simulink model "Solar_Seguidor_V2"  (R2021b)
settings: Solver=ode1  StartTime=0.0  StopTime=10  FixedStep=25e-6  RelTol=1e-3
PostLoadFcn:
  | %clc; clear all; close all;
  | %%%%%%%%%%%%%%%%%%%%%%%%%%%%%%%%%%%%%%%%%%%%%%%%
  | %%%%%%%%% Solar seguidor de rede %%%%%%%%%%
  | %%%%%%%%%%%%%%%%%%%%%%%%%%%%%%%%%%%%%%%%%%%%%%%%
  | %%%% Nominal Parameters %%%%
  | Pnom = 16e3;                                         % Potencia Nominal
  | Vnom_rms = 210;                                    % V linha rms
  | Vnom_peak = sqrt(2/3)*Vnom_rms;                     % V fase pico
  | FP_min = 1;                                       % Para suporte de reativo
  | Snom = Pnom/FP_min;                                 % Potencia aparente
  | Irms = Pnom/(sqrt(3)*Vnom_rms);                     % Ig rms
  | Inom_peak = Irms*sqrt(2);                           % Ig pico
  | Zbase = Vnom_peak/Inom_peak;                        % Impedancia Base
  | f = 60;                                             % Freq nominal
  | wnom = 2*pi*60;                                     % Freq Ang. nominal
  | m = 0.805;                                            % Indice mod nominal
  | Vdc = 2*(Vnom_peak/m);                              % Vcc
  | Vdc_2 = Vdc/2;                                      % Metade Vcc
  | Kconv = Zbase;                                      % Ganho conversor
  | %%%% Transformer %%%%
  | S_trafo = 250e3;                                      % transformer apparent power
  | Vrms_high = 400;                                   % transformer secondary voltage - Wye connection
  | Vrms_low = 210;                                   % transformer primary voltage - Delta connection
  | N = Vrms_high/Vrms_low;                             % transformation relationship
  | X_pu_trafo = 0.03;                                 % transformer p.u. reactance
  | Zb_trafo_high = ((Vrms_high)^2)/S_trafo;            % secondary base impedance
  | Zb_trafo = ((Vnom_rms)^2)/S_trafo;                  % primary base impedance
  | L_trafo = (X_pu_trafo*Zb_trafo)/wnom;               % primary inductance
  | %%%% LCL Filter Project %%%%
  | fsw = 105*60;%105*60;                                         % switching frequency
  | ripple = 0.05;                                       % current ripple
  | L1 = Vdc/(6*ripple*Inom_peak*fsw);                  % inductor L1
  |  RL1 = 0.005;                                        % L1 resistance
  |  Cbase = 1/(wnom*Kconv);                             % base capacitance
  |  Cf = 0.05*Cbase;                                    % filter capacitor
  | % Calculo do filtro
  | Sbase = 16e3;
  | %Sbase = 200e3*1.12;
  | V_LL = 210;
  | V_LG = 210/sqrt(3);
  | Vbase = V_LG*sqrt(2);
  | Ibase = (Sbase*sqrt(2))/(V_LG*3)*sqrt(3/2);
  | Zbase = (V_LL^2)/Sbase;
  | Rbase = Zbase;
  | Xbase = Zbase;
  | Lbase = Xbase/(2*pi*60);
  | Cbase = 1/(Xbase*2*pi*60);
  | w = 2*pi*60;
  | Q = 70;
  | Lf = 0.15*Lbase;
  | Cf = 0.05*Cbase;
  | fc = 1/(2*pi*sqrt(Lf*Cf));
  | R = (w*Lf)/Q;
  | Lf = L1;
  | R = RL1;
  | ka=0.2;                                             % attenuation factor
  | L2 = (sqrt(1/(ka^2))+1)/(Cf*((2*pi*fsw)^2));        % inductor L2
  | RL2 = 0.005;                                        % L2 resistance
  | w_res = sqrt((L1+L2+L_trafo)/(L1*L2*Cf));           % resonant angular frequency
  | f_res = w_res/(2*pi);                               % resonant frequency
  | ... (+31 lines)
InitFcn:
  | %clc; clear all; close all;
  | %%%%%%%%%%%%%%%%%%%%%%%%%%%%%%%%%%%%%%%%%%%%%%%%
  | %%%%%%%%% Solar seguidor de rede %%%%%%%%%%
  | %%%%%%%%%%%%%%%%%%%%%%%%%%%%%%%%%%%%%%%%%%%%%%%%
  | %%%% Nominal Parameters %%%%
  | Pnom = 16e3;                                         % Potencia Nominal
  | Vnom_rms = 210;                                    % V linha rms
  | Vnom_peak = sqrt(2/3)*Vnom_rms;                     % V fase pico
  | FP_min = 1;                                       % Para suporte de reativo
  | Snom = Pnom/FP_min;                                 % Potencia aparente
  | Irms = Pnom/(sqrt(3)*Vnom_rms);                     % Ig rms
  | Inom_peak = Irms*sqrt(2);                           % Ig pico
  | Zbase = Vnom_peak/Inom_peak;                        % Impedancia Base
  | f = 60;                                             % Freq nominal
  | wnom = 2*pi*60;                                     % Freq Ang. nominal
  | m = 0.805;                                            % Indice mod nominal
  | Vdc = 2*(Vnom_peak/m);                              % Vcc
  | Vdc_2 = Vdc/2;                                      % Metade Vcc
  | Kconv = Zbase;                                      % Ganho conversor
  | %%%% Transformer %%%%
  | S_trafo = 250e3;                                      % transformer apparent power
  | Vrms_high = 400;                                   % transformer secondary voltage - Wye connection
  | Vrms_low = 210;                                   % transformer primary voltage - Delta connection
  | N = Vrms_high/Vrms_low;                             % transformation relationship
  | X_pu_trafo = 0.03;                                 % transformer p.u. reactance
  | Zb_trafo_high = ((Vrms_high)^2)/S_trafo;            % secondary base impedance
  | Zb_trafo = ((Vnom_rms)^2)/S_trafo;                  % primary base impedance
  | L_trafo = (X_pu_trafo*Zb_trafo)/wnom;               % primary inductance
  | %%%% LCL Filter Project %%%%
  | fsw = 105*60;%105*60;                                         % switching frequency
  | ripple = 0.05;                                       % current ripple
  | L1 = Vdc/(6*ripple*Inom_peak*fsw);                  % inductor L1
  |  RL1 = 0.005;                                        % L1 resistance
  |  Cbase = 1/(wnom*Kconv);                             % base capacitance
  |  Cf = 0.05*Cbase;                                    % filter capacitor
  | % Calculo do filtro
  | Sbase = 16e3;
  | %Sbase = 200e3*1.12;
  | V_LL = 210;
  | V_LG = 210/sqrt(3);
  | Vbase = V_LG*sqrt(2);
  | Ibase = (Sbase*sqrt(2))/(V_LG*3)*sqrt(3/2);
  | Zbase = (V_LL^2)/Sbase;
  | Rbase = Zbase;
  | Xbase = Zbase;
  | Lbase = Xbase/(2*pi*60);
  | Cbase = 1/(Xbase*2*pi*60);
  | w = 2*pi*60;
  | Q = 70;
  | Lf = 0.15*Lbase;
  | Cf = 0.05*Cbase;
  | fc = 1/(2*pi*sqrt(Lf*Cf));
  | R = (w*Lf)/Q;
  | Lf = L1;
  | R = RL1;
  | ka=0.2;                                             % attenuation factor
  | L2 = (sqrt(1/(ka^2))+1)/(Cf*((2*pi*fsw)^2));        % inductor L2
  | RL2 = 0.005;                                        % L2 resistance
  | w_res = sqrt((L1+L2+L_trafo)/(L1*L2*Cf));           % resonant angular frequency
  | f_res = w_res/(2*pi);                               % resonant frequency
  | ... (+31 lines)
undefined symbols (not defined in the file): D1, Delta, DERS_models, DiscIntNeverNeededParam, eHS, I, Ia_PV, Ib_PV, Ic_PV, Left, parameter_set_id, ph, PV_system, type, V, Va_grid, Vb_grid, Vc_grid
libraries: powerlib_meascontrol x17, rtlab x14, spsThreePhaseSeriesRLCBranchLib x9, spsCurrentMeasurementLib x9, artemis x7, spsThreePhaseVIMeasurementLib x6, slpidlib x6, rteventslib x6, spsabctodq0Lib x4, spsThreePhaseTransformerTwoWindingsLib x3, simulink x3, spsPVArrayLib x3
(part 3 of 4)

== system Solar_Seguidor_V2/SM_mestre1/PV_system/Subsystem1/THD ==
  Iabc : Inport
  Demux : Demux  Outputs=3
  Gain1 : Gain  Gain=100
  Gain2 : Gain  Gain=100
  Gain3 : Gain  Gain=100
  Mux : Mux  Inputs=3
  Saturation : Saturate  UpperLimit=7
  Saturation1 : Saturate  UpperLimit=7
  Saturation2 : Saturate  UpperLimit=7
  THD : powerlib_meascontrol/Measurements/THD  Freq=60  Ts=Ts
  THD1 : powerlib_meascontrol/Measurements/THD  Freq=60  Ts=Ts
  THD2 : powerlib_meascontrol/Measurements/THD  Freq=60  Ts=Ts
  THD_I : Outport
  wires:
  Demux/1 -> THD/1
  Saturation2/1 -> Mux/3
  Saturation/1 -> Mux/1
  THD/1 -> Gain1/1
  Saturation1/1 -> Mux/2
  Demux/3 -> THD2/1
  THD1/1 -> Gain2/1
  Gain2/1 -> Saturation1/1
  Gain3/1 -> Saturation2/1
  THD2/1 -> Gain3/1
  Demux/2 -> THD1/1
  Gain1/1 -> Saturation/1
  Iabc/1 -> Demux/1
  Mux/1 -> THD_I/1

== system Solar_Seguidor_V2/SM_mestre1/PV_system/VSC_Control/Current Controller ==
  note: Current Controller (with feedforward)
  VdVq_mes : Inport  PortDimensions=2
  IdIq_mes : Inport  Port=2  PortDimensions=2
  IdIq_ref : Inport  Port=3  PortDimensions=2
  hab : Inport  Port=4
  Add1 : Sum  Inputs=+-
  Add2 : Sum
  Add3 : Sum
  Demux : Demux  Outputs=2
  Demux1 : Demux  Outputs=2
  Mux : Mux  Inputs=2
  Mux1 : Mux  Inputs=2
  PI : slpidlib/PID Controller  Controller=PI  Form=Parallel  TimeDomain=Continuous-time  UseExternalTs=off  SampleTime=Ts  IntegratorMethod=Forward Euler  FilterMethod=Forward Euler  ControllerParametersSource=internal  P=kp_current_pu  I=ki_current_pu  D=0  UseFilter=on  N=100  TunerSelectOption=Transfer Function Based (PID Tuner App)  InitialConditionSource=internal  InitialConditionForIntegrator=0  InitialConditionForFilter=0  DifferentiatorICPrevScaledInput=0  ExternalReset=rising  TrackingMode=off  Kt=1  LimitOutput=off  SatLimitsSource=internal  UpperSaturationLimit=2  LowerSaturationLimit=-2  LinearizeAsGain=off  AntiWindupMode=none  Kb=1  POutMin=[]  POutMax=[]  IOutMin=[]  IOutMax=[]  DOutMin=[]  DOutMax=[]  NOutMin=[]  NOutMax=[]  SumOutMin=[]  SumOutMax=[]  SaturationOutMin=[]  SaturationOutMax=[]  PParamMin=[]  PParamMax=[]  IParamMin=[]  IParamMax=[]  DParamMin=[]  DParamMax=[]  NParamMin=[]  NParamMax=[]  KbParamMin=[]  KbParamMax=[]  KtParamMin=[]  KtParamMax=[]  KbOutMin=[]  KbOutMax=[]  KtOutMin=[]  KtOutMax=[]  IntegratorOutMin=[]  IntegratorOutMax=[]  FilterOutMin=[]  FilterOutMax=[]  SumI1OutMin=[]  SumI1OutMax=[]  SumI2OutMin=[]  SumI2OutMax=[]  SumI3OutMin=[]  SumI3OutMax=[]  SumI4OutMin=[]  SumI4OutMax=[]  SumDOutMin=[]  SumDOutMax=[]  DifferentiatorOutMin=[]  DifferentiatorOutMax=[]  FilterDiffOutCoefMin=[]  FilterDiffOutCoefMax=[]  ReciprocalOutMin=[]  ReciprocalOutMax=[]  SumDenOutMin=[]  SumDenOutMax=[]  SumNumOutMin=[]  SumNumOutMax=[]  DivideOutMin=[]  DivideOutMax=[]  UdiffTsProdOutMin=[]  UdiffTsProdOutMax=[]  NTsProdOutMin=[]  NTsProdOutMax=[]  UintegralTsProdOutMin=[]  UintegralTsProdOutMax=[]  UngainTsProdOutMin=[]  UngainTsProdOutMax=[]  IntegratorContinuousStateAttributes=''  IntegratorStateMustResolveToSignalObject=off  IntegratorRTWStateStorageClass=Auto  FilterContinuousStateAttributes=''  FilterStateMustResolveToSignalObject=off  FilterRTWStateStorageClass=Auto  ParallelPVariant=InternalParameters  IdealPVariant=Disabled  IVariant=InternalParameters  DVariant=Disabled  IntegratorVariant=Continuous  SatVariant=Disabled  AWVariant=Passthrough  PCopyVariant=Disabled  TRVariant=Disabled  FdbkBlocksVariant=Forward  IdealPFdbkVariant=Disabled  SatFdbkVariant=Disabled  DerivativeFilterVariant=Disabled  NVariant=Disabled  NCopyVariant=Disabled_SignalSpec  FilterICVariant=Disabled  IntegratorICVariant=InternalICs  ExternalResetVariant=ExternalReset  TRSumVariant=Passthrough  SumFdbkVariant=Disabled  SumVariant=Sum_PI  TsampFilterVariant=InternalTs  TsampNgainVariant=Passthrough  TsampIntegralVariant=Passthrough  ExternalSaturationOutDataTypeStr=Inherit: Same as second input
  Product : Product
  Saturation : Saturate  UpperLimit=10  LowerLimit=-10
  Sum : Sum  Inputs=|+-
  wL : Gain  Gain=decouple_pu  SaturateOnIntegerOverflow=on  OutDataTypeStr=Inherit: Same as input  ParamDataTypeStr=Inherit: Same as input
  wL2 : Gain  Gain=decouple_pu  SaturateOnIntegerOverflow=on  OutDataTypeStr=Inherit: Same as input  ParamDataTypeStr=Inherit: Same as input
  m_dq : Outport  VectorParamsAs1DForOutWhenUnconnected=off
  wires:
  wL/1 -> Add1/2
  Mux/1 -> Add2/2
  PI/1 -> Add2/1  "PI"
  Sum/1 -> PI/1
  Saturation/1 -> m_dq/1
  VdVq_mes/1 -> Demux/1
  Demux/1 -> Add1/1
  Demux1/1 -> wL2/1
  Demux1/2 -> wL/1
  wL2/1 -> Add3/2
  Add1/1 -> Mux/1
  Demux/2 -> Add3/1
  Add3/1 -> Mux/2
  Add2/1 -> Product/1
  Product/1 -> Saturation/1
  hab/1 -> [hab]
  [hab] -> PI/2
  [hab] -> Product/2
  Mux1/1 -> [Idq_scope]
  IdIq_ref/1 -> Mux1/1, Sum/1
  IdIq_mes/1 -> Mux1/2, Sum/2, Demux1/1

== system Solar_Seguidor_V2/SM_mestre1/PV_system/VSC_Control/Maximum Power Point ==
  Vpv : Inport
  Ipv : Inport  Port=2
  Enable_MPPT : Inport  Port=3
  Constant : Constant  Value=Vdc
  MPPT Parameters : Subsystem
  MPPT Controller using Perturbe & Observe technique 2 : MATLAB Function  TreatAsAtomicUnit=on
  Switch1 : Switch
  ZOH/4 : ZeroOrderHold  SampleTime=Ts_Control
  ZOH/6 : ZeroOrderHold  SampleTime=Ts_Control
  Gmpp : Outport
  wires:
  Ipv/1 -> ZOH/6/1
  Vpv/1 -> ZOH/4/1
  ZOH/4/1 -> MPPT Controller using Perturbe & Observe technique 2/3(V)
  ZOH/6/1 -> MPPT Controller using Perturbe & Observe technique 2/4(I)
  MPPT Parameters/1(Param) -> MPPT Controller using Perturbe & Observe technique 2/1(Param)
  Enable_MPPT/1 -> MPPT Controller using Perturbe & Observe technique 2/2(Enabled), Switch1/2
  Constant/1 -> Switch1/3
  Switch1/1 -> Gmpp/1
  MPPT Controller using Perturbe & Observe technique 2/1(D) -> Switch1/1

== system Solar_Seguidor_V2/SM_mestre1/PV_system/VSC_Control/PLL & dq ==
  Vabc : Inport
  Iabc : Inport  Port=2
  Demux : Demux  Outputs=2
  I_to_pu : Gain  Gain=1/(Ibase*1.15)  SaturateOnIntegerOverflow=on  OutDataTypeStr=Inherit: Same as input  ParamDataTypeStr=Inherit: Same as input
  Iabc_PV : Scope
  Iabc_PV_pu : Scope
  Idq : Scope
  Mux1 : Mux  Inputs=2
  PLL (3ph) : powerlib_meascontrol/PLL/PLL (3ph)  Fmin=45  Par_Init="[-0.57  60]"  ParK=[180, 3200, 1]  TcD=Ts_Control  MaxRateChangeFreq=12  FilterCutOffFreq=25  Ts=Ts_Control  AGC=on
  Scope : Scope
  Scope1 : Scope
  Selector1 : Selector  InputPortWidth=3  IndexOptions=Index vector (dialog)  Indices=[1 2]  OutputSizes=1
  Selector2 : Selector  InputPortWidth=3  IndexOptions=Index vector (dialog)  Indices=[1 2]  OutputSizes=1
  Subsystem : Subsystem
  Transfer Fcn1 : TransferFcn  Denominator=[2.53e-4 1]
  Transfer Fcn4 : TransferFcn  Denominator=[2.53e-4 1]
  V_to_pu : Gain  Gain=1/(400*sqrt(2)/sqrt(3))  SaturateOnIntegerOverflow=on  OutDataTypeStr=Inherit: Same as input  ParamDataTypeStr=Inherit: Same as input
  abc to dq0 : powerlib_meascontrol/Transformations/abc to dq0  Alignment=90 degrees behind phase A axis
  abc to dq1 : powerlib_meascontrol/Transformations/abc to dq0  Alignment=90 degrees behind phase A axis
  P_PV : Outport
  Freq : Outport  Port=2
  wt : Outport  Port=3  VectorParamsAs1DForOutWhenUnconnected=off
  VdVq : Outport  Port=4  VectorParamsAs1DForOutWhenUnconnected=off
  IdIq : Outport  Port=5  VectorParamsAs1DForOutWhenUnconnected=off
  wires:
  Iabc/1 -> Iabc_PV/1, Subsystem/3(Iabc), I_to_pu/1
  I_to_pu/1 -> Iabc_PV_pu/1, abc to dq1/1
  V_to_pu/1 -> abc to dq0/1, PLL (3ph)/1
  abc to dq1/1 -> Selector1/1
  Vabc/1 -> Subsystem/2(Vabc), V_to_pu/1
  abc to dq0/1 -> Selector2/1
  PLL (3ph)/1 -> Scope1/1, Freq/1
  Selector1/1 -> Demux/1
  Demux/1 -> Transfer Fcn4/1
  Demux/2 -> Transfer Fcn1/1
  Mux1/1 -> Idq/1, IdIq/1
  Selector2/1 -> Scope/1, VdVq/1
  Subsystem/1(P_PV) -> P_PV/1
  PLL (3ph)/2 -> Subsystem/1(wt), abc to dq1/2, abc to dq0/2, wt/1
  Transfer Fcn4/1 -> Mux1/1
  Transfer Fcn1/1 -> Mux1/2

== system Solar_Seguidor_V2/SM_mestre1/PV_system/VSC_Control/PWM ==
  Uabc_ref : Inport
  Constant10 : Constant  Value=2
  Constant11 : Constant  Value=3*35*60
  Constant9 : Constant
  Demux8 : Demux  Outputs=3
  Divide7 : Product  Inputs=*/
  Divide8 : Product  Inputs=*/
  Divide9 : Product  Inputs=*/
  Mux11 : Mux  Inputs=3
  Mux12 : Mux  Inputs=2
  RTE Conversion1 : rteventslib/Signal Attributes/RTE Conversion  inputdatatype=RTE Boolean  outputdatatype=Double  compensation=Enabled  nbMaxEvents=4  sampleTime=Ts
  RTE SPWM1 : rteventslib/Sources/RTE SPWM  NumberPhases=3-ph  CenterAlignmentMode=On  MaxFreq=inf  MinFreq=0  EnablingPort=off  ComplementaryMode=on  SpaceVector=off  RiseTimeDelay=0  MaxEvents=4  SampleTime=Ts
  Saturation : Saturate  UpperLimit=2  LowerLimit=-2
  Scope : Scope
  Scope8 : Scope
  Selector1 : Selector  InputPortWidth=6  IndexOptions=Index vector (dialog)  Indices=[1 4 2 5 3 6]  OutputSizes=1
  Sum16 : Sum  Inputs=|++
  Sum17 : Sum  Inputs=|++
  Sum18 : Sum  Inputs=|++
  Uref : Outport  VectorParamsAs1DForOutWhenUnconnected=off
  wires:
  RTE Conversion1/1 -> Selector1/1
  Mux12/1 -> RTE Conversion1/1
  Demux8/3 -> Sum18/1
  Demux8/1 -> Sum16/1
  Divide7/1 -> Mux11/1
  Mux11/1 -> Scope8/1, RTE SPWM1/2
  Sum18/1 -> Divide9/1
  Divide8/1 -> Mux11/2
  Demux8/2 -> Sum17/1
  Uabc_ref/1 -> Saturation/1
  RTE SPWM1/2 -> Mux12/2
  Divide9/1 -> Mux11/3
  Sum17/1 -> Divide8/1
  Constant10/1 -> Divide7/2, Divide8/2, Divide9/2
  Sum16/1 -> Divide7/1
  Constant11/1 -> RTE SPWM1/1
  Selector1/1 -> Uref/1
  Constant9/1 -> Sum16/2, Sum17/2, Sum18/2
  RTE SPWM1/1 -> Mux12/1
  Saturation/1 -> Scope/1, Demux8/1

== system Solar_Seguidor_V2/SM_mestre1/PV_system/VSC_Control/Uabc_ref Generation  ==
  note: Uabc_ref Generation
  wt : Inport
  m_dq : Inport  Port=2
  Constant5 : Constant  Value=0
  Mux : Mux  Inputs=2
  Scope : Scope
  dq0 to abc : spsdq0toabcLib/dq0 to abc  Alignment=90 degrees behind phase A axis
  Uabc_ref : Outport  VectorParamsAs1DForOutWhenUnconnected=off
  wires:
  Mux/1 -> dq0 to abc/1
  Constant5/1 -> Mux/2
  wt/1 -> dq0 to abc/2
  dq0 to abc/1 -> Uabc_ref/1
  m_dq/1 -> Scope/1, Mux/1

== system Solar_Seguidor_V2/SM_mestre1/PV_system/VSC_Control/Voltage DC Controller ==
  note: Voltage Controller
  Vdc_mes : Inport  PortDimensions=1
  Vdc_ref : Inport  Port=2  PortDimensions=1
  hab : Inport  Port=3
  Id_refm : Scope
  Math Function1 : Math  Operator=square  SaturateOnIntegerOverflow=on
  Math Function2 : Math  Commented=on  Operator=square  SaturateOnIntegerOverflow=on
  Math Function3 : Math  Operator=square  SaturateOnIntegerOverflow=on
  Mux : Mux  Inputs=2
  PI : slpidlib/PID Controller  Controller=PI  Form=Parallel  TimeDomain=Continuous-time  UseExternalTs=off  SampleTime=Ts  IntegratorMethod=Trapezoidal  FilterMethod=Forward Euler  ControllerParametersSource=internal  P=Kp_dc  I=ki_dc_pu  D=0  UseFilter=on  N=100  TunerSelectOption=Transfer Function Based (PID Tuner App)  InitialConditionSource=internal  InitialConditionForIntegrator=0  InitialConditionForFilter=0  DifferentiatorICPrevScaledInput=0  ExternalReset=rising  TrackingMode=off  Kt=1  LimitOutput=on  SatLimitsSource=internal  UpperSaturationLimit=1.4  LowerSaturationLimit=-2  LinearizeAsGain=off  AntiWindupMode=clamping  Kb=1  POutMin=[]  POutMax=[]  IOutMin=[]  IOutMax=[]  DOutMin=[]  DOutMax=[]  NOutMin=[]  NOutMax=[]  SumOutMin=[]  SumOutMax=[]  SaturationOutMin=[]  SaturationOutMax=[]  PParamMin=[]  PParamMax=[]  IParamMin=[]  IParamMax=[]  DParamMin=[]  DParamMax=[]  NParamMin=[]  NParamMax=[]  KbParamMin=[]  KbParamMax=[]  KtParamMin=[]  KtParamMax=[]  KbOutMin=[]  KbOutMax=[]  KtOutMin=[]  KtOutMax=[]  IntegratorOutMin=[]  IntegratorOutMax=[]  FilterOutMin=[]  FilterOutMax=[]  SumI1OutMin=[]  SumI1OutMax=[]  SumI2OutMin=[]  SumI2OutMax=[]  SumI3OutMin=[]  SumI3OutMax=[]  SumI4OutMin=[]  SumI4OutMax=[]  SumDOutMin=[]  SumDOutMax=[]  DifferentiatorOutMin=[]  DifferentiatorOutMax=[]  FilterDiffOutCoefMin=[]  FilterDiffOutCoefMax=[]  ReciprocalOutMin=[]  ReciprocalOutMax=[]  SumDenOutMin=[]  SumDenOutMax=[]  SumNumOutMin=[]  SumNumOutMax=[]  DivideOutMin=[]  DivideOutMax=[]  UdiffTsProdOutMin=[]  UdiffTsProdOutMax=[]  NTsProdOutMin=[]  NTsProdOutMax=[]  UintegralTsProdOutMin=[]  UintegralTsProdOutMax=[]  UngainTsProdOutMin=[]  UngainTsProdOutMax=[]  IntegratorContinuousStateAttributes=''  IntegratorStateMustResolveToSignalObject=off  IntegratorRTWStateStorageClass=Auto  FilterContinuousStateAttributes=''  FilterStateMustResolveToSignalObject=off  FilterRTWStateStorageClass=Auto  ParallelPVariant=InternalParameters  IdealPVariant=Disabled  IVariant=InternalParameters  DVariant=Disabled  IntegratorVariant=Continuous  SatVariant=Enabled  AWVariant=ContClampingParallel  PCopyVariant=Disabled  TRVariant=Disabled  FdbkBlocksVariant=Forward  IdealPFdbkVariant=Disabled  SatFdbkVariant=Disabled  DerivativeFilterVariant=Disabled  NVariant=Disabled  NCopyVariant=Disabled_SignalSpec  FilterICVariant=Disabled  IntegratorICVariant=InternalICs  ExternalResetVariant=ExternalReset  TRSumVariant=Passthrough  SumFdbkVariant=Disabled  SumVariant=Sum_PI  TsampFilterVariant=InternalTs  TsampNgainVariant=Passthrough  TsampIntegralVariant=Passthrough  ExternalSaturationOutDataTypeStr=Inherit: Same as second input
  Rtot_pu1 : Gain  Gain=1/430  SaturateOnIntegerOverflow=on  OutDataTypeStr=Inherit: Same as input  ParamDataTypeStr=Inherit: Same as input
  Rtot_pu2 : Gain  Gain=1/430  SaturateOnIntegerOverflow=on  OutDataTypeStr=Inherit: Same as input  ParamDataTypeStr=Inherit: Same as input
  Rtot_pu3 : Gain  Gain=-1  SaturateOnIntegerOverflow=on  OutDataTypeStr=Inherit: Same as input  ParamDataTypeStr=Inherit: Same as input
  Saturation : Saturate  UpperLimit=1.2  LowerLimit=0
  Sum : Sum  Inputs=|-+
  Transfer Fcn2 : TransferFcn  Commented=on  Denominator=[2.53e-4 1]
  Id_ref : Outport  SampleTime=Ts  InitialOutput=0  VectorParamsAs1DForOutWhenUnconnected=off
  wires:
  Rtot_pu3/1 -> PI/1
  Vdc_ref/1 -> Rtot_pu2/1
  Sum/1 -> Rtot_pu3/1
  hab/1 -> PI/2
  Mux/1 -> [Vdc_scope]
  Rtot_pu1/1 -> Mux/1, Math Function1/1
  Rtot_pu2/1 -> Mux/2, Math Function3/1
  Math Function1/1 -> Sum/1
  Math Function3/1 -> Sum/2
  PI/1 -> Id_refm/1, Saturation/1
  Vdc_mes/1 -> Rtot_pu1/1
  Saturation/1 -> Id_ref/1

== system Solar_Seguidor_V2/SM_mestre1/PV_system1/Subsystem1/THD ==
  Iabc : Inport
  Demux : Demux  Outputs=3
  Gain1 : Gain  Gain=100
  Gain2 : Gain  Gain=100
  Gain3 : Gain  Gain=100
  Mux : Mux  Inputs=3
  Saturation : Saturate  UpperLimit=7
  Saturation1 : Saturate  UpperLimit=7
  Saturation2 : Saturate  UpperLimit=7
  THD : powerlib_meascontrol/Measurements/THD  Freq=60  Ts=Ts
  THD1 : powerlib_meascontrol/Measurements/THD  Freq=60  Ts=Ts
  THD2 : powerlib_meascontrol/Measurements/THD  Freq=60  Ts=Ts
  THD_I : Outport
  wires:
  Mux/1 -> THD_I/1
  Iabc/1 -> Demux/1
  Gain1/1 -> Saturation/1
  Demux/2 -> THD1/1
  THD2/1 -> Gain3/1
  Gain3/1 -> Saturation2/1
  Gain2/1 -> Saturation1/1
  THD1/1 -> Gain2/1
  Demux/3 -> THD2/1
  Saturation1/1 -> Mux/2
  THD/1 -> Gain1/1
  Saturation/1 -> Mux/1
  Saturation2/1 -> Mux/3
  Demux/1 -> THD/1

== system Solar_Seguidor_V2/SM_mestre1/PV_system1/VSC_Control/Current Controller ==
  note: Current Controller (with feedforward)
  VdVq_mes : Inport  PortDimensions=2
  IdIq_mes : Inport  Port=2  PortDimensions=2
  IdIq_ref : Inport  Port=3  PortDimensions=2
  hab : Inport  Port=4
  Add1 : Sum  Inputs=+-
  Add2 : Sum
  Add3 : Sum
  Demux : Demux  Outputs=2
  Demux1 : Demux  Outputs=2
  Mux : Mux  Inputs=2
  Mux1 : Mux  Inputs=2
  PI : slpidlib/PID Controller  Controller=PI  Form=Parallel  TimeDomain=Continuous-time  UseExternalTs=off  SampleTime=Ts  IntegratorMethod=Forward Euler  FilterMethod=Forward Euler  ControllerParametersSource=internal  P=kp_current_pu  I=ki_current_pu  D=0  UseFilter=on  N=100  TunerSelectOption=Transfer Function Based (PID Tuner App)  InitialConditionSource=internal  InitialConditionForIntegrator=0  InitialConditionForFilter=0  DifferentiatorICPrevScaledInput=0  ExternalReset=rising  TrackingMode=off  Kt=1  LimitOutput=off  SatLimitsSource=internal  UpperSaturationLimit=2  LowerSaturationLimit=-2  LinearizeAsGain=off  AntiWindupMode=none  Kb=1  POutMin=[]  POutMax=[]  IOutMin=[]  IOutMax=[]  DOutMin=[]  DOutMax=[]  NOutMin=[]  NOutMax=[]  SumOutMin=[]  SumOutMax=[]  SaturationOutMin=[]  SaturationOutMax=[]  PParamMin=[]  PParamMax=[]  IParamMin=[]  IParamMax=[]  DParamMin=[]  DParamMax=[]  NParamMin=[]  NParamMax=[]  KbParamMin=[]  KbParamMax=[]  KtParamMin=[]  KtParamMax=[]  KbOutMin=[]  KbOutMax=[]  KtOutMin=[]  KtOutMax=[]  IntegratorOutMin=[]  IntegratorOutMax=[]  FilterOutMin=[]  FilterOutMax=[]  SumI1OutMin=[]  SumI1OutMax=[]  SumI2OutMin=[]  SumI2OutMax=[]  SumI3OutMin=[]  SumI3OutMax=[]  SumI4OutMin=[]  SumI4OutMax=[]  SumDOutMin=[]  SumDOutMax=[]  DifferentiatorOutMin=[]  DifferentiatorOutMax=[]  FilterDiffOutCoefMin=[]  FilterDiffOutCoefMax=[]  ReciprocalOutMin=[]  ReciprocalOutMax=[]  SumDenOutMin=[]  SumDenOutMax=[]  SumNumOutMin=[]  SumNumOutMax=[]  DivideOutMin=[]  DivideOutMax=[]  UdiffTsProdOutMin=[]  UdiffTsProdOutMax=[]  NTsProdOutMin=[]  NTsProdOutMax=[]  UintegralTsProdOutMin=[]  UintegralTsProdOutMax=[]  UngainTsProdOutMin=[]  UngainTsProdOutMax=[]  FilterDenConstantOutDataTypeStr=Inherit: Inherit via back propagation  FilterDenConstantOutMin=[]  FilterDenConstantOutMax=[]  PCopyOutDataTypeStr=Inherit: Inherit via back propagation  PCopyOutMin=[]  PCopyOutMax=[]  NCopyOutDataTypeStr=Inherit: Inherit via back propagation  NCopyOutMin=[]  NCopyOutMax=[]  IntegratorContinuousStateAttributes=''  IntegratorStateMustResolveToSignalObject=off  IntegratorRTWStateStorageClass=Auto  FilterContinuousStateAttributes=''  FilterStateMustResolveToSignalObject=off  FilterRTWStateStorageClass=Auto  ParallelPVariant=InternalParameters  IdealPVariant=Disabled  IVariant=InternalParameters  DVariant=Disabled  IntegratorVariant=Continuous  SatVariant=Disabled  AWVariant=Passthrough  PCopyVariant=Disabled  TRVariant=Disabled  FdbkBlocksVariant=Forward  IdealPFdbkVariant=Disabled  SatFdbkVariant=Disabled  DerivativeFilterVariant=Disabled  NVariant=Disabled  NCopyVariant=Disabled_SignalSpec  FilterICVariant=Disabled  IntegratorICVariant=InternalICs  ExternalResetVariant=ExternalReset  TRSumVariant=Passthrough  SumFdbkVariant=Disabled  SumVariant=Sum_PI  TsampFilterVariant=InternalTs  TsampNgainVariant=Passthrough  TsampIntegralVariant=Passthrough  ExternalSaturationOutDataTypeStr=Inherit: Same as second input
  Product : Product
  Saturation : Saturate  UpperLimit=10  LowerLimit=-10
  Sum : Sum  Inputs=|+-
  wL : Gain  Gain=decouple_pu  SaturateOnIntegerOverflow=on  OutDataTypeStr=Inherit: Same as input  ParamDataTypeStr=Inherit: Same as input
  wL2 : Gain  Gain=decouple_pu  SaturateOnIntegerOverflow=on  OutDataTypeStr=Inherit: Same as input  ParamDataTypeStr=Inherit: Same as input
  m_dq : Outport  VectorParamsAs1DForOutWhenUnconnected=off
  wires:
  IdIq_mes/1 -> Demux1/1, Sum/2, Mux1/2
  IdIq_ref/1 -> Sum/1, Mux1/1
  Mux1/1 -> [Idq_scope]
  [hab] -> Product/2
  [hab] -> PI/2
  hab/1 -> [hab]
  Product/1 -> Saturation/1
  Add2/1 -> Product/1
  Add3/1 -> Mux/2
  Demux/2 -> Add3/1
  Add1/1 -> Mux/1
  wL2/1 -> Add3/2
  Demux1/2 -> wL/1
  Demux1/1 -> wL2/1
  Demux/1 -> Add1/1
  VdVq_mes/1 -> Demux/1
  Saturation/1 -> m_dq/1
  Sum/1 -> PI/1
  PI/1 -> Add2/1  "PI"
  Mux/1 -> Add2/2
  wL/1 -> Add1/2

== system Solar_Seguidor_V2/SM_mestre1/PV_system1/VSC_Control/Maximum Power Point ==
  Vpv : Inport
  Ipv : Inport  Port=2
  Enable_MPPT : Inport  Port=3
  Constant : Constant  Value=Vdc
  MPPT Parameters : Subsystem
  MPPT Controller using Perturbe & Observe technique 2 : MATLAB Function  TreatAsAtomicUnit=on
  Switch1 : Switch
  ZOH/4 : ZeroOrderHold  SampleTime=Ts_Control
  ZOH/6 : ZeroOrderHold  SampleTime=Ts_Control
  Gmpp : Outport
  wires:
  MPPT Controller using Perturbe & Observe technique 2/1(D) -> Switch1/1
  Switch1/1 -> Gmpp/1
  Constant/1 -> Switch1/3
  Enable_MPPT/1 -> Switch1/2, MPPT Controller using Perturbe & Observe technique 2/2(Enabled)
  MPPT Parameters/1(Param) -> MPPT Controller using Perturbe & Observe technique 2/1(Param)
  ZOH/6/1 -> MPPT Controller using Perturbe & Observe technique 2/4(I)
  ZOH/4/1 -> MPPT Controller using Perturbe & Observe technique 2/3(V)
  Vpv/1 -> ZOH/4/1
  Ipv/1 -> ZOH/6/1

== system Solar_Seguidor_V2/SM_mestre1/PV_system1/VSC_Control/PLL & dq ==
  Vabc : Inport
  Iabc : Inport  Port=2
  Demux : Demux  Outputs=2
  I_to_pu : Gain  Gain=1/(Ibase*1.15)  SaturateOnIntegerOverflow=on  OutDataTypeStr=Inherit: Same as input  ParamDataTypeStr=Inherit: Same as input
  Iabc_PV : Scope
  Iabc_PV_pu : Scope
  Idq : Scope
  Mux1 : Mux  Inputs=2
  PLL (3ph) : powerlib_meascontrol/PLL/PLL (3ph)  Fmin=45  Par_Init="[-0.57  60]"  ParK=[180, 3200, 1]  TcD=Ts_Control  MaxRateChangeFreq=12  FilterCutOffFreq=25  Ts=Ts_Control  AGC=on
  Scope : Scope
  Scope1 : Scope
  Selector1 : Selector  InputPortWidth=3  IndexOptions=Index vector (dialog)  Indices=[1 2]  OutputSizes=1
  Selector2 : Selector  InputPortWidth=3  IndexOptions=Index vector (dialog)  Indices=[1 2]  OutputSizes=1
  Subsystem : Subsystem
  Transfer Fcn1 : TransferFcn  Denominator=[2.53e-4 1]
  Transfer Fcn4 : TransferFcn  Denominator=[2.53e-4 1]
  V_to_pu : Gain  Gain=1/(400*sqrt(2)/sqrt(3))  SaturateOnIntegerOverflow=on  OutDataTypeStr=Inherit: Same as input  ParamDataTypeStr=Inherit: Same as input
  abc to dq0 : powerlib_meascontrol/Transformations/abc to dq0  Alignment=90 degrees behind phase A axis
  abc to dq1 : powerlib_meascontrol/Transformations/abc to dq0  Alignment=90 degrees behind phase A axis
  P_PV : Outport
  Freq : Outport  Port=2
  wt : Outport  Port=3  VectorParamsAs1DForOutWhenUnconnected=off
  VdVq : Outport  Port=4  VectorParamsAs1DForOutWhenUnconnected=off
  IdIq : Outport  Port=5  VectorParamsAs1DForOutWhenUnconnected=off
  wires:
  Transfer Fcn1/1 -> Mux1/2
  Transfer Fcn4/1 -> Mux1/1
  PLL (3ph)/2 -> wt/1, abc to dq0/2, abc to dq1/2, Subsystem/1(wt)
  Subsystem/1(P_PV) -> P_PV/1
  Selector2/1 -> VdVq/1, Scope/1
  Mux1/1 -> IdIq/1, Idq/1
  Demux/2 -> Transfer Fcn1/1
  Demux/1 -> Transfer Fcn4/1
  Selector1/1 -> Demux/1
  PLL (3ph)/1 -> Freq/1, Scope1/1
  abc to dq0/1 -> Selector2/1
  Vabc/1 -> V_to_pu/1, Subsystem/2(Vabc)
  abc to dq1/1 -> Selector1/1
  V_to_pu/1 -> PLL (3ph)/1, abc to dq0/1
  I_to_pu/1 -> abc to dq1/1, Iabc_PV_pu/1
  Iabc/1 -> I_to_pu/1, Subsystem/3(Iabc), Iabc_PV/1

== system Solar_Seguidor_V2/SM_mestre1/PV_system1/VSC_Control/PWM ==
  Uabc_ref : Inport
  Constant10 : Constant  Value=2
  Constant11 : Constant  Value=3*35*60
  Constant9 : Constant
  Demux8 : Demux  Outputs=3
  Divide7 : Product  Inputs=*/
  Divide8 : Product  Inputs=*/
  Divide9 : Product  Inputs=*/
  Mux11 : Mux  Inputs=3
  Mux12 : Mux  Inputs=2
  RTE Conversion1 : rteventslib/Signal Attributes/RTE Conversion  inputdatatype=RTE Boolean  outputdatatype=Double  compensation=Enabled  nbMaxEvents=4  sampleTime=Ts
  RTE SPWM1 : rteventslib/Sources/RTE SPWM  NumberPhases=3-ph  CenterAlignmentMode=On  MaxFreq=inf  MinFreq=0  EnablingPort=off  ComplementaryMode=on  SpaceVector=off  RiseTimeDelay=0  MaxEvents=4  SampleTime=Ts
  Saturation : Saturate  UpperLimit=2  LowerLimit=-2
  Scope : Scope
  Scope8 : Scope
  Selector1 : Selector  InputPortWidth=6  IndexOptions=Index vector (dialog)  Indices=[1 4 2 5 3 6]  OutputSizes=1
  Sum16 : Sum  Inputs=|++
  Sum17 : Sum  Inputs=|++
  Sum18 : Sum  Inputs=|++
  Uref : Outport  VectorParamsAs1DForOutWhenUnconnected=off
  wires:
  Saturation/1 -> Demux8/1, Scope/1
  RTE SPWM1/1 -> Mux12/1
  Constant9/1 -> Sum18/2, Sum17/2, Sum16/2
  Selector1/1 -> Uref/1
  Constant11/1 -> RTE SPWM1/1
  Sum16/1 -> Divide7/1
  Constant10/1 -> Divide9/2, Divide8/2, Divide7/2
  Sum17/1 -> Divide8/1
  Divide9/1 -> Mux11/3
  RTE SPWM1/2 -> Mux12/2
  Uabc_ref/1 -> Saturation/1
  Demux8/2 -> Sum17/1
  Divide8/1 -> Mux11/2
  Sum18/1 -> Divide9/1
  Mux11/1 -> RTE SPWM1/2, Scope8/1
  Divide7/1 -> Mux11/1
  Demux8/1 -> Sum16/1
  Demux8/3 -> Sum18/1
  Mux12/1 -> RTE Conversion1/1
  RTE Conversion1/1 -> Selector1/1

== system Solar_Seguidor_V2/SM_mestre1/PV_system1/VSC_Control/Uabc_ref Generation  ==
  note: Uabc_ref Generation
  wt : Inport
  m_dq : Inport  Port=2
  Constant5 : Constant  Value=0
  Mux : Mux  Inputs=2
  Scope : Scope
  dq0 to abc : spsdq0toabcLib/dq0 to abc  Alignment=90 degrees behind phase A axis
  Uabc_ref : Outport  VectorParamsAs1DForOutWhenUnconnected=off
  wires:
  m_dq/1 -> Mux/1, Scope/1
  dq0 to abc/1 -> Uabc_ref/1
  wt/1 -> dq0 to abc/2
  Constant5/1 -> Mux/2
  Mux/1 -> dq0 to abc/1

== system Solar_Seguidor_V2/SM_mestre1/PV_system1/VSC_Control/Voltage DC Controller ==
  note: Voltage Controller
  Vdc_mes : Inport  PortDimensions=1
  Vdc_ref : Inport  Port=2  PortDimensions=1
  hab : Inport  Port=3
  Id_refm : Scope
  Math Function1 : Math  Operator=square  SaturateOnIntegerOverflow=on
  Math Function2 : Math  Commented=on  Operator=square  SaturateOnIntegerOverflow=on
  Math Function3 : Math  Operator=square  SaturateOnIntegerOverflow=on
  Mux : Mux  Inputs=2
  PI : slpidlib/PID Controller  Controller=PI  Form=Parallel  TimeDomain=Continuous-time  UseExternalTs=off  SampleTime=Ts  IntegratorMethod=Trapezoidal  FilterMethod=Forward Euler  ControllerParametersSource=internal  P=Kp_dc  I=ki_dc_pu  D=0  UseFilter=on  N=100  TunerSelectOption=Transfer Function Based (PID Tuner App)  InitialConditionSource=internal  InitialConditionForIntegrator=0  InitialConditionForFilter=0  DifferentiatorICPrevScaledInput=0  ExternalReset=rising  TrackingMode=off  Kt=1  LimitOutput=on  SatLimitsSource=internal  UpperSaturationLimit=1.4  LowerSaturationLimit=-2  LinearizeAsGain=off  AntiWindupMode=clamping  Kb=1  POutMin=[]  POutMax=[]  IOutMin=[]  IOutMax=[]  DOutMin=[]  DOutMax=[]  NOutMin=[]  NOutMax=[]  SumOutMin=[]  SumOutMax=[]  SaturationOutMin=[]  SaturationOutMax=[]  PParamMin=[]  PParamMax=[]  IParamMin=[]  IParamMax=[]  DParamMin=[]  DParamMax=[]  NParamMin=[]  NParamMax=[]  KbParamMin=[]  KbParamMax=[]  KtParamMin=[]  KtParamMax=[]  KbOutMin=[]  KbOutMax=[]  KtOutMin=[]  KtOutMax=[]  IntegratorOutMin=[]  IntegratorOutMax=[]  FilterOutMin=[]  FilterOutMax=[]  SumI1OutMin=[]  SumI1OutMax=[]  SumI2OutMin=[]  SumI2OutMax=[]  SumI3OutMin=[]  SumI3OutMax=[]  SumI4OutMin=[]  SumI4OutMax=[]  SumDOutMin=[]  SumDOutMax=[]  DifferentiatorOutMin=[]  DifferentiatorOutMax=[]  FilterDiffOutCoefMin=[]  FilterDiffOutCoefMax=[]  ReciprocalOutMin=[]  ReciprocalOutMax=[]  SumDenOutMin=[]  SumDenOutMax=[]  SumNumOutMin=[]  SumNumOutMax=[]  DivideOutMin=[]  DivideOutMax=[]  UdiffTsProdOutMin=[]  UdiffTsProdOutMax=[]  NTsProdOutMin=[]  NTsProdOutMax=[]  UintegralTsProdOutMin=[]  UintegralTsProdOutMax=[]  UngainTsProdOutMin=[]  UngainTsProdOutMax=[]  FilterDenConstantOutDataTypeStr=Inherit: Inherit via back propagation  FilterDenConstantOutMin=[]  FilterDenConstantOutMax=[]  PCopyOutDataTypeStr=Inherit: Inherit via back propagation  PCopyOutMin=[]  PCopyOutMax=[]  NCopyOutDataTypeStr=Inherit: Inherit via back propagation  NCopyOutMin=[]  NCopyOutMax=[]  IntegratorContinuousStateAttributes=''  IntegratorStateMustResolveToSignalObject=off  IntegratorRTWStateStorageClass=Auto  FilterContinuousStateAttributes=''  FilterStateMustResolveToSignalObject=off  FilterRTWStateStorageClass=Auto  ParallelPVariant=InternalParameters  IdealPVariant=Disabled  IVariant=InternalParameters  DVariant=Disabled  IntegratorVariant=Continuous  SatVariant=Enabled  AWVariant=ContClampingParallel  PCopyVariant=Disabled  TRVariant=Disabled  FdbkBlocksVariant=Forward  IdealPFdbkVariant=Disabled  SatFdbkVariant=Disabled  DerivativeFilterVariant=Disabled  NVariant=Disabled  NCopyVariant=Disabled_SignalSpec  FilterICVariant=Disabled  IntegratorICVariant=InternalICs  ExternalResetVariant=ExternalReset  TRSumVariant=Passthrough  SumFdbkVariant=Disabled  SumVariant=Sum_PI  TsampFilterVariant=InternalTs  TsampNgainVariant=Passthrough  TsampIntegralVariant=Passthrough  ExternalSaturationOutDataTypeStr=Inherit: Same as second input
  Rtot_pu1 : Gain  Gain=1/430  SaturateOnIntegerOverflow=on  OutDataTypeStr=Inherit: Same as input  ParamDataTypeStr=Inherit: Same as input
  Rtot_pu2 : Gain  Gain=1/430  SaturateOnIntegerOverflow=on  OutDataTypeStr=Inherit: Same as input  ParamDataTypeStr=Inherit: Same as input
  Rtot_pu3 : Gain  Gain=-1  SaturateOnIntegerOverflow=on  OutDataTypeStr=Inherit: Same as input  ParamDataTypeStr=Inherit: Same as input
  Saturation : Saturate  UpperLimit=1.2  LowerLimit=0
  Sum : Sum  Inputs=|-+
  Transfer Fcn2 : TransferFcn  Commented=on  Denominator=[2.53e-4 1]
  Id_ref : Outport  SampleTime=Ts  InitialOutput=0  VectorParamsAs1DForOutWhenUnconnected=off
  wires:
  Saturation/1 -> Id_ref/1
  Vdc_mes/1 -> Rtot_pu1/1
  PI/1 -> Saturation/1, Id_refm/1
  Math Function3/1 -> Sum/2
  Math Function1/1 -> Sum/1
  Rtot_pu2/1 -> Math Function3/1, Mux/2
  Rtot_pu1/1 -> Math Function1/1, Mux/1
  Mux/1 -> [Vdc_scope]
  hab/1 -> PI/2
  Sum/1 -> Rtot_pu3/1
  Vdc_ref/1 -> Rtot_pu2/1
  Rtot_pu3/1 -> PI/1

== system Solar_Seguidor_V2/SM_mestre1/PV_system2/Subsystem1/THD ==
  Iabc : Inport
  Demux : Demux  Outputs=3
  Gain1 : Gain  Gain=100
  Gain2 : Gain  Gain=100
  Gain3 : Gain  Gain=100
  Mux : Mux  Inputs=3
  Saturation : Saturate  UpperLimit=7
  Saturation1 : Saturate  UpperLimit=7
  Saturation2 : Saturate  UpperLimit=7
  THD : spsTHDLib/THD  Freq=60  Ts=Ts
      settings: SourceProductBaseCode=PS
  THD1 : spsTHDLib/THD  Freq=60  Ts=Ts
      settings: SourceProductBaseCode=PS
  THD2 : spsTHDLib/THD  Freq=60  Ts=Ts
      settings: SourceProductBaseCode=PS
  THD_I : Outport
  wires:
  Mux/1 -> THD_I/1
  Iabc/1 -> Demux/1
  Gain1/1 -> Saturation/1
  Demux/2 -> THD1/1
  THD2/1 -> Gain3/1
  Gain3/1 -> Saturation2/1
  Gain2/1 -> Saturation1/1
  THD1/1 -> Gain2/1
  Demux/3 -> THD2/1
  Saturation1/1 -> Mux/2
  THD/1 -> Gain1/1
  Saturation/1 -> Mux/1
  Saturation2/1 -> Mux/3
  Demux/1 -> THD/1

== system Solar_Seguidor_V2/SM_mestre1/PV_system2/VSC_Control/Current Controller ==
  note: Current Controller (with feedforward)
  VdVq_mes : Inport  PortDimensions=2
  IdIq_mes : Inport  Port=2  PortDimensions=2
  IdIq_ref : Inport  Port=3  PortDimensions=2
  hab : Inport  Port=4
  Add1 : Sum  Inputs=+-
  Add2 : Sum
  Add3 : Sum
  Demux : Demux  Outputs=2
  Demux1 : Demux  Outputs=2
  Idq : Scope
  Mux : Mux  Inputs=2
  Mux1 : Mux  Inputs=2
  PI : slpidlib/PID Controller  Commented=on  Controller=PI  Form=Parallel  TimeDomain=Continuous-time  UseExternalTs=off  SampleTime=Ts  IntegratorMethod=Forward Euler  FilterMethod=Forward Euler  ControllerParametersSource=internal  P=kp_current_pu  I=ki_current_pu  D=0  UseFilter=on  N=100  TunerSelectOption=Transfer Function Based (PID Tuner App)  InitialConditionSource=internal  InitialConditionForIntegrator=0  InitialConditionForFilter=0  DifferentiatorICPrevScaledInput=0  ExternalReset=rising  TrackingMode=off  Kt=1  LimitOutput=off  SatLimitsSource=internal  UpperSaturationLimit=2  LowerSaturationLimit=-2  LinearizeAsGain=off  AntiWindupMode=none  Kb=1  POutMin=[]  POutMax=[]  IOutMin=[]  IOutMax=[]  DOutMin=[]  DOutMax=[]  NOutMin=[]  NOutMax=[]  SumOutMin=[]  SumOutMax=[]  SaturationOutMin=[]  SaturationOutMax=[]  PParamMin=[]  PParamMax=[]  IParamMin=[]  IParamMax=[]  DParamMin=[]  DParamMax=[]  NParamMin=[]  NParamMax=[]  KbParamMin=[]  KbParamMax=[]  KtParamMin=[]  KtParamMax=[]  KbOutMin=[]  KbOutMax=[]  KtOutMin=[]  KtOutMax=[]  IntegratorOutMin=[]  IntegratorOutMax=[]  FilterOutMin=[]  FilterOutMax=[]  SumI1OutMin=[]  SumI1OutMax=[]  SumI2OutMin=[]  SumI2OutMax=[]  SumI3OutMin=[]  SumI3OutMax=[]  SumI4OutMin=[]  SumI4OutMax=[]  SumDOutMin=[]  SumDOutMax=[]  DifferentiatorOutMin=[]  DifferentiatorOutMax=[]  FilterDiffOutCoefMin=[]  FilterDiffOutCoefMax=[]  ReciprocalOutMin=[]  ReciprocalOutMax=[]  SumDenOutMin=[]  SumDenOutMax=[]  SumNumOutMin=[]  SumNumOutMax=[]  DivideOutMin=[]  DivideOutMax=[]  UdiffTsProdOutMin=[]  UdiffTsProdOutMax=[]  NTsProdOutMin=[]  NTsProdOutMax=[]  UintegralTsProdOutMin=[]  UintegralTsProdOutMax=[]  UngainTsProdOutMin=[]  UngainTsProdOutMax=[]  FilterDenConstantOutDataTypeStr=Inherit: Inherit via back propagation  FilterDenConstantOutMin=[]  FilterDenConstantOutMax=[]  PCopyOutDataTypeStr=Inherit: Inherit via back propagation  PCopyOutMin=[]  PCopyOutMax=[]  NCopyOutDataTypeStr=Inherit: Inherit via back propagation  NCopyOutMin=[]  NCopyOutMax=[]  IntegratorContinuousStateAttributes=''  IntegratorStateMustResolveToSignalObject=off  IntegratorRTWStateStorageClass=Auto  FilterContinuousStateAttributes=''  FilterStateMustResolveToSignalObject=off  FilterRTWStateStorageClass=Auto  ParallelPVariant=InternalParameters  IdealPVariant=Disabled  IVariant=InternalParameters  DVariant=Disabled  IntegratorVariant=Continuous  SatVariant=Disabled  AWVariant=Passthrough  PCopyVariant=Disabled  TRVariant=Disabled  FdbkBlocksVariant=Forward  IdealPFdbkVariant=Disabled  SatFdbkVariant=Disabled  DerivativeFilterVariant=Disabled  NVariant=Disabled  NCopyVariant=Disabled_SignalSpec  FilterICVariant=Disabled  IntegratorICVariant=InternalICs  ExternalResetVariant=ExternalReset  TRSumVariant=Passthrough  SumFdbkVariant=Disabled  SumVariant=Sum_PI  TsampFilterVariant=InternalTs  TsampNgainVariant=Passthrough  TsampIntegralVariant=Passthrough  ExternalSaturationOutDataTypeStr=Inherit: Same as second input
  PI_Idq1 : Subsystem
  Product : Product
  Saturation : Saturate  UpperLimit=10  LowerLimit=-10
  Sum : Sum  Inputs=|+-
  wL : Gain  Gain=decouple_pu  SaturateOnIntegerOverflow=on  OutDataTypeStr=Inherit: Same as input  ParamDataTypeStr=Inherit: Same as input
  wL2 : Gain  Gain=decouple_pu  SaturateOnIntegerOverflow=on  OutDataTypeStr=Inherit: Same as input  ParamDataTypeStr=Inherit: Same as input
  m_dq : Outport  VectorParamsAs1DForOutWhenUnconnected=off
  wires:
  IdIq_mes/1 -> Demux1/1, Sum/2, Mux1/2
  IdIq_ref/1 -> Sum/1, Mux1/1
  Mux1/1 -> [Idq_scope], Idq/1
  [hab] -> Product/2
  [hab] -> PI_Idq1/2(hab)
  hab/1 -> [hab]
  Product/1 -> Saturation/1
  Add2/1 -> Product/1
  Add3/1 -> Mux/2
  Demux/2 -> Add3/1
  Add1/1 -> Mux/1
  wL2/1 -> Add3/2
  Demux1/2 -> wL/1
  Demux1/1 -> wL2/1
  Demux/1 -> Add1/1
  VdVq_mes/1 -> Demux/1
  Saturation/1 -> m_dq/1
  Sum/1 -> PI_Idq1/1(e_Idq)
  PI_Idq1/1(u) -> Add2/1  "PI"
  Mux/1 -> Add2/2
  wL/1 -> Add1/2

== system Solar_Seguidor_V2/SM_mestre1/PV_system2/VSC_Control/Maximum Power Point ==
  Vpv : Inport
  Ipv : Inport  Port=2
  Enable_MPPT : Inport  Port=3
  Constant : Constant  Value=Vdc
  MPPT Parameters : Subsystem
  MPPT Controller using Perturbe & Observe technique 2 : MATLAB Function  TreatAsAtomicUnit=on
  Switch1 : Switch
  ZOH/4 : ZeroOrderHold  SampleTime=Ts_Control
  ZOH/6 : ZeroOrderHold  SampleTime=Ts_Control
  Gmpp : Outport
  wires:
  MPPT Controller using Perturbe & Observe technique 2/1(D) -> Switch1/1
  Switch1/1 -> Gmpp/1
  Constant/1 -> Switch1/3
  Enable_MPPT/1 -> Switch1/2, MPPT Controller using Perturbe & Observe technique 2/2(Enabled)
  MPPT Parameters/1(Param) -> MPPT Controller using Perturbe & Observe technique 2/1(Param)
  ZOH/6/1 -> MPPT Controller using Perturbe & Observe technique 2/4(I)
  ZOH/4/1 -> MPPT Controller using Perturbe & Observe technique 2/3(V)
  Vpv/1 -> ZOH/4/1
  Ipv/1 -> ZOH/6/1

== system Solar_Seguidor_V2/SM_mestre1/PV_system2/VSC_Control/PLL & dq ==
  Vabc : Inport
  Iabc : Inport  Port=2
  Demux : Demux  Outputs=2
  I_to_pu : Gain  Gain=1/(Ibase*1.25)  SaturateOnIntegerOverflow=on  OutDataTypeStr=Inherit: Same as input  ParamDataTypeStr=Inherit: Same as input
  Iabc_PV : Scope
  Iabc_PV_pu : Scope
  Idq : Scope
  Mux1 : Mux  Inputs=2
  PLL (3ph) : spsPLL3phLib/PLL (3ph)  Fmin=45  Par_Init="[-0.57  60]"  ParK=[180, 3200, 1]  TcD=Ts_Control  MaxRateChangeFreq=12  FilterCutOffFreq=25  Ts=Ts_Control  AGC=on
  Scope : Scope
  Scope1 : Scope
  Selector1 : Selector  InputPortWidth=3  IndexOptions=Index vector (dialog)  Indices=[1 2]  OutputSizes=1
  Selector2 : Selector  InputPortWidth=3  IndexOptions=Index vector (dialog)  Indices=[1 2]  OutputSizes=1
  Subsystem : Subsystem
  Transfer Fcn1 : TransferFcn  Denominator=[2.53e-4 1]
  Transfer Fcn4 : TransferFcn  Denominator=[2.53e-4 1]
  V_to_pu : Gain  Gain=1/(400*sqrt(2)/sqrt(3))  SaturateOnIntegerOverflow=on  OutDataTypeStr=Inherit: Same as input  ParamDataTypeStr=Inherit: Same as input
  abc to dq0 : spsabctodq0Lib/abc to dq0  Alignment=90 degrees behind phase A axis
  abc to dq1 : spsabctodq0Lib/abc to dq0  Alignment=90 degrees behind phase A axis
  P_PV : Outport
  Freq : Outport  Port=2
  wt : Outport  Port=3  VectorParamsAs1DForOutWhenUnconnected=off
  VdVq : Outport  Port=4  VectorParamsAs1DForOutWhenUnconnected=off
  IdIq : Outport  Port=5  VectorParamsAs1DForOutWhenUnconnected=off
  wires:
  Transfer Fcn1/1 -> Mux1/2
  Transfer Fcn4/1 -> Mux1/1
  PLL (3ph)/2 -> wt/1, abc to dq0/2, abc to dq1/2, Subsystem/1(wt)
  Subsystem/1(P_PV) -> P_PV/1
  Selector2/1 -> VdVq/1, Scope/1
  Mux1/1 -> IdIq/1, Idq/1
  Demux/2 -> Transfer Fcn1/1
  Demux/1 -> Transfer Fcn4/1
  Selector1/1 -> Demux/1
  PLL (3ph)/1 -> Freq/1, Scope1/1
  abc to dq0/1 -> Selector2/1
  Vabc/1 -> V_to_pu/1, Subsystem/2(Vabc)
  abc to dq1/1 -> Selector1/1
  V_to_pu/1 -> PLL (3ph)/1, abc to dq0/1
  I_to_pu/1 -> abc to dq1/1, Iabc_PV_pu/1
  Iabc/1 -> I_to_pu/1, Subsystem/3(Iabc), Iabc_PV/1

== system Solar_Seguidor_V2/SM_mestre1/PV_system2/VSC_Control/PWM ==
  Uabc_ref : Inport
  Constant10 : Constant  Value=2
  Constant11 : Constant  Value=3*35*60
  Constant9 : Constant
  Demux8 : Demux  Outputs=3
  Divide7 : Product  Inputs=*/
  Divide8 : Product  Inputs=*/
  Divide9 : Product  Inputs=*/
  Mux11 : Mux  Inputs=3
  Mux12 : Mux  Inputs=2
  RTE Conversion1 : rteventslib/Signal Attributes/RTE Conversion  inputdatatype=RTE Boolean  outputdatatype=Double  compensation=Enabled  nbMaxEvents=4  sampleTime=Ts
  RTE SPWM1 : rteventslib/Sources/RTE SPWM  NumberPhases=3-ph  CenterAlignmentMode=On  MaxFreq=inf  MinFreq=0  EnablingPort=off  ComplementaryMode=on  SpaceVector=off  RiseTimeDelay=0  MaxEvents=4  SampleTime=Ts
  Saturation : Saturate  UpperLimit=2  LowerLimit=-2
  Scope : Scope
  Scope8 : Scope
  Selector1 : Selector  InputPortWidth=6  IndexOptions=Index vector (dialog)  Indices=[1 4 2 5 3 6]  OutputSizes=1
  Sum16 : Sum  Inputs=|++
  Sum17 : Sum  Inputs=|++
  Sum18 : Sum  Inputs=|++
  Uref : Outport  VectorParamsAs1DForOutWhenUnconnected=off
  wires:
  Saturation/1 -> Demux8/1, Scope/1
  RTE SPWM1/1 -> Mux12/1
  Constant9/1 -> Sum18/2, Sum17/2, Sum16/2
  Selector1/1 -> Uref/1
  Constant11/1 -> RTE SPWM1/1
  Sum16/1 -> Divide7/1
  Constant10/1 -> Divide9/2, Divide8/2, Divide7/2
  Sum17/1 -> Divide8/1
  Divide9/1 -> Mux11/3
  RTE SPWM1/2 -> Mux12/2
  Uabc_ref/1 -> Saturation/1
  Demux8/2 -> Sum17/1
  Divide8/1 -> Mux11/2
  Sum18/1 -> Divide9/1
  Mux11/1 -> RTE SPWM1/2, Scope8/1
  Divide7/1 -> Mux11/1
  Demux8/1 -> Sum16/1
  Demux8/3 -> Sum18/1
  Mux12/1 -> RTE Conversion1/1
  RTE Conversion1/1 -> Selector1/1

== system Solar_Seguidor_V2/SM_mestre1/PV_system2/VSC_Control/Uabc_ref Generation  ==
  note: Uabc_ref Generation
  wt : Inport
  m_dq : Inport  Port=2
  Constant5 : Constant  Value=0
  Mux : Mux  Inputs=2
  Scope : Scope
  dq0 to abc : spsdq0toabcLib/dq0 to abc  Alignment=90 degrees behind phase A axis
  Uabc_ref : Outport  VectorParamsAs1DForOutWhenUnconnected=off
  wires:
  m_dq/1 -> Mux/1, Scope/1
  dq0 to abc/1 -> Uabc_ref/1
  wt/1 -> dq0 to abc/2
  Constant5/1 -> Mux/2
  Mux/1 -> dq0 to abc/1
